simulink model "Model2"  (R2019b)
settings: Solver=VariableStepAuto  StartTime=0.0  StopTime=time  FixedStep=0.01  RelTol=1e-3
values from neighbouring files (symbols this model uses):
  breath = 60/f    (= 3)    [Model_main.m]
  E1 = 16    [Model_main.m]
  E_th = 5    [Model_main.m]
  insptime = (ieratio(1)/(ieratio(1)+ieratio(2)))*100    [Model_main.m]
  Pcontrol = 15    [Model_main.m]
  PEEP = 5    [Model_main.m]
  R1 = 15    [Model_main.m]
  V0 = 2    [Model_main.m]
  V0_th = 4.6    [Model_main.m]
settings Model: Creator=Amne  LastModifiedBy=Amne
settings DataIOCC: ReturnWorkspaceOutputsName=SDOSimTest_Log
settings DebuggingCC: ArithmeticOperatorsInVariantConditions=warning
settings SFSimCC: SimUseLocalCustomCode=off  CustomCodeUndefinedFunction=UseInterfaceOnly
settings RTWCC: RTWUseLocalCustomCode=off

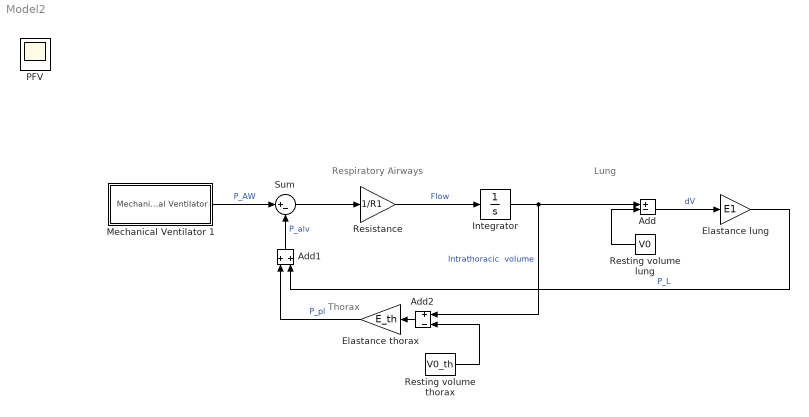
== system Model2 ==
  note: Thorax
  note: Lung
  note: Respiratory Airways
  Add : Sum  Inputs=+-
  Add1 : Sum
  Add2 : Sum  Inputs=+-
  Elastance lung : Gain  Gain=E1
  Elastance thorax : Gain  Gain=E_th
  Integrator : Integrator  ZeroCross=off
  Mechanical Ventilator 1 : Subsystem
  Resistance : Gain  Gain=1/R1
  Resting volume lung : Constant  Value=V0
  Resting volume thorax : Constant  Value=V0_th
  Sum : Sum  Inputs=|+-
  PFV : Scope
  wires:
  Integrator/1 -> Add2/1, Add/1  "Intrathoracic  volume"
  Elastance lung/1 -> Add1/2  "P_L"
  Resistance/1 -> Integrator/1  "Flow"
  Sum/1 -> Resistance/1
  Add/1 -> Elastance lung/1  "dV"
  Resting volume lung/1 -> Add/2
  Mechanical Ventilator 1/1(Mechanical Ventilator) -> Sum/1  "P_AW"
  Elastance thorax/1 -> Add1/1  "P_pl"
  Add1/1 -> Sum/2  "P_alv"
  Resting volume thorax/1 -> Add2/2
  Add2/1 -> Elastance thorax/1

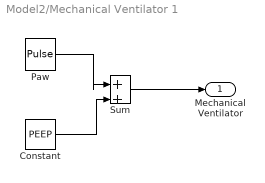
== system Model2/Mechanical Ventilator 1 ==
  Constant : Constant  Value=PEEP  SampleTime=0.1
  Paw : DiscretePulseGenerator  PulseType=Time based  Amplitude=Pcontrol  Period=breath  PulseWidth=insptime  PhaseDelay=2  SampleTime=0.1
  Sum : Sum  Inputs=|++
  Mechanical Ventilator : Outport  VectorParamsAs1DForOutWhenUnconnected=off
  wires:
  Paw/1 -> Sum/1
  Constant/1 -> Sum/2
  Sum/1 -> Mechanical Ventilator/1
